simulink model "silnik"  (R2018b)
settings: Solver=ode4  StartTime=0.0  StopTime=100.0  FixedStep=0.001  RelTol=1e-3
values from neighbouring files (symbols this model uses):
  A = 1.8    [dane.m]
  B = 0.0002    [dane.m]
  C = 0.3    [dane.m]
  g = 9.81    [dane.m]
  G = 11    [dane.m]
  J = 0.05    [dane.m]
  Laf = 6.008e-3    (= 0.006008)    [dane.m]
  LaiLfield = 1.766e-3    (= 0.001766)    [dane.m]
  m = 800    [dane.m]
  mirr = 0.015    [dane.m]
  r = 0.25    [dane.m]
  RaiRf = 0.12    [dane.m]
  ro = 1.25    [dane.m]
settings Model: Creator=lpa2  LastModifiedBy=Sonia
settings SFSimCC: SimUseLocalCustomCode=off
settings RTWCC: RTWUseLocalCustomCode=off

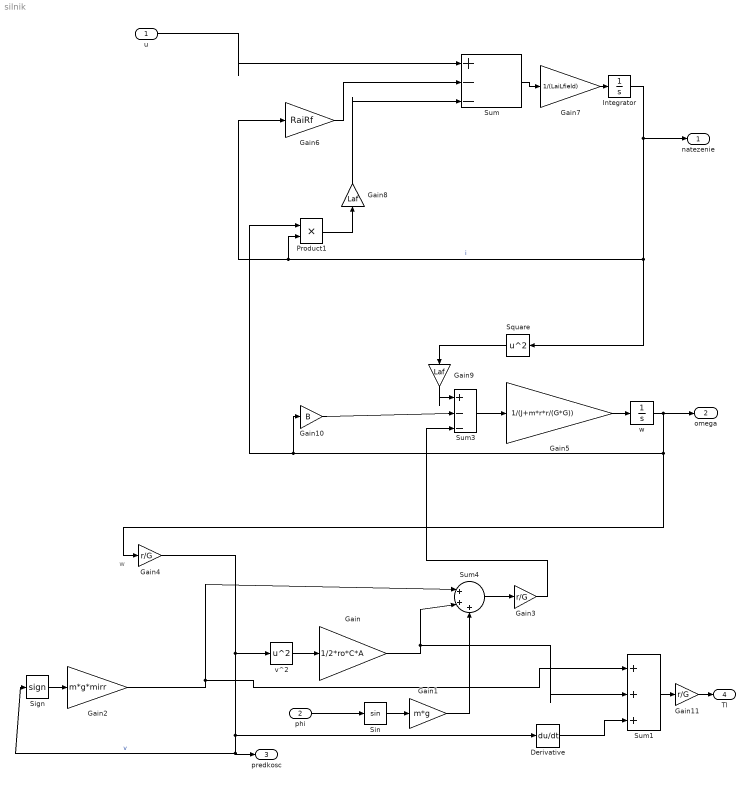
== system silnik ==
  note: w
  u : Inport
  phi : Inport  Port=2
  Derivative : Derivative
  Gain : Gain  Gain=1/2*ro*C*A
  Gain1 : Gain  Gain=m*g
  Gain10 : Gain  Gain=B
  Gain11 : Gain  Gain=r/G
  Gain2 : Gain  Gain=m*g*mirr
  Gain3 : Gain  Gain=r/G
  Gain4 : Gain  Gain=r/G
  Gain5 : Gain  Gain=1/(J+m*r*r/(G*G))
  Gain6 : Gain  Gain=RaiRf
  Gain7 : Gain  Gain=1/(LaiLfield)
  Gain8 : Gain  Gain=Laf
  Gain9 : Gain  Gain=Laf
  Integrator : Integrator
  Product1 : Product
  Sign : Signum
  Sin : Trigonometry
  Square : Math  Operator=square  RndMeth=Zero  SaturateOnIntegerOverflow=on
  Sum : Sum  Inputs=|+--
  Sum1 : Sum  Inputs=|+++
  Sum3 : Sum  Inputs=|+--
  Sum4 : Sum  Inputs=|+++
  v^2 : Math  Operator=square  RndMeth=Zero  SaturateOnIntegerOverflow=on
  w : Integrator
  natezenie : Outport
  omega : Outport  Port=2
  predkosc : Outport  Port=3
  Tl : Outport  Port=4
  wires:
  u/1 -> Sum/1
  Gain6/1 -> Sum/2
  Sum/1 -> Gain7/1
  Gain7/1 -> Integrator/1
  Integrator/1 -> natezenie/1, Gain6/1, Product1/2, Square/1  "i"
  Gain9/1 -> Sum3/1
  Square/1 -> Gain9/1
  Gain10/1 -> Sum3/2
  Gain4/1 -> Derivative/1, predkosc/1, Sign/1, v^2/1  "v"
  v^2/1 -> Gain/1
  Gain/1 -> Sum1/2, Sum4/2
  phi/1 -> Sin/1
  Sin/1 -> Gain1/1
  Gain1/1 -> Sum4/3
  Sign/1 -> Gain2/1
  Sum4/1 -> Gain3/1
  Gain3/1 -> Sum3/3
  Sum3/1 -> Gain5/1
  Gain5/1 -> w/1
  w/1 -> Gain10/1, Product1/1, Gain4/1, omega/1
  Product1/1 -> Gain8/1
  Gain8/1 -> Sum/3
  Gain2/1 -> Sum1/1, Sum4/1
  Derivative/1 -> Sum1/3
  Sum1/1 -> Gain11/1
  Gain11/1 -> Tl/1
